simulink model "arq11"  (R2013a)
settings: Solver=ode45  StartTime=0.0  StopTime=Tsim  RelTol=1e-3
values from neighbouring files (symbols this model uses):
  D = 4.1019    [load_variables.m]    (also in matlab.mat; matlab2.mat; matlab_workspace.mat)
  dist = 0    [Ensaios_artigo.m]    (also in load_variables.m = 5; matlab.mat = 5; matlab2.mat = 5; matlab_workspace.mat = 5)
  gain_reduce = 0.9    [Ensaios_artigo.m]
  I = 0.0044    [load_variables.m]    (also in matlab.mat; matlab2.mat; matlab_workspace.mat)
  P = 0.3105    [load_variables.m]    (also in matlab.mat; matlab2.mat; matlab_workspace.mat)
  ref = 10    [Ensaios_artigo.m]    (also in load_variables.m; matlab.mat; matlab2.mat; matlab_workspace.mat)
  Tdist = 0    [Ensaios_artigo.m]    (also in RenameVar.m = Tstep; matlab.mat = 1200; matlab2.mat = 1200; matlab_workspace.mat = 1400)
  Tdistdown = 0    [Ensaios_artigo.m]    (also in RenameVar.m = Tstepdown; matlab.mat = 1800; matlab2.mat = 1800; matlab_workspace.mat = 1800)
  Tref = 700    [Ensaios_artigo.m]    (also in load_variables.m = 800; matlab.mat = 600; matlab2.mat = 600; matlab_workspace.mat)
  Trefdown = Tref*2    (= 1400)    [Ensaios_artigo.m]    (also in load_variables.m = 2420; matlab.mat = 2400; matlab2.mat = 2400; matlab_workspace.mat = 2500)
  Ts = 5    [load_variables.m]    (also in matlab.mat; matlab2.mat; matlab_workspace.mat)
  Tsim = Tref+Trefdown    (= 2100)    [Ensaios_artigo.m]    (also in load_variables.m = 3220; matlab.mat = 800; matlab2.mat = 800; matlab_workspace.mat = 3200)
undefined symbols (not defined in the file): sigma_n, Td
libraries: cstblocks x5, opclib x3, simulink x2, commchan3 x1
settings Model: Creator=didaticontrol  LastModifiedBy=didaticontrol

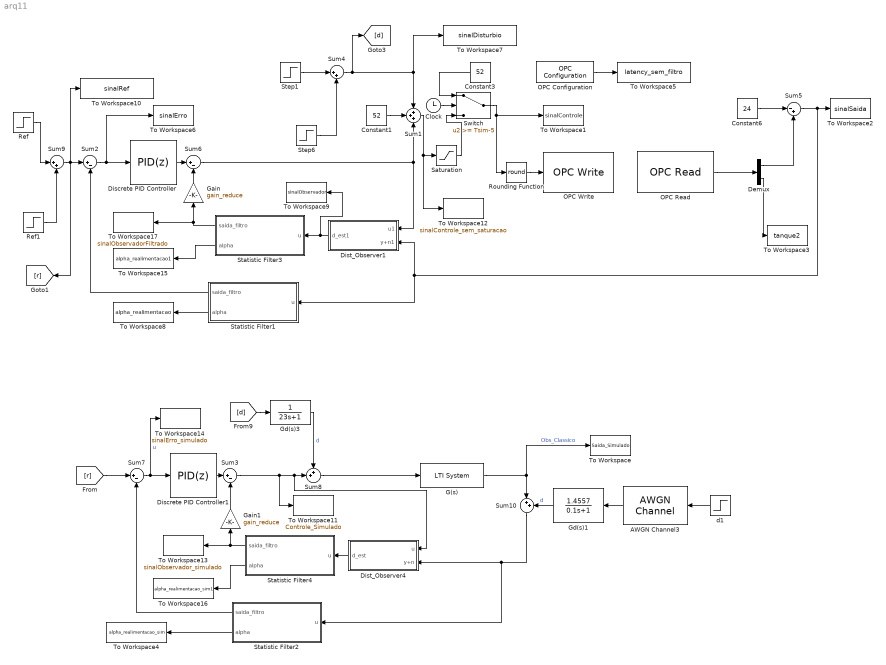
== system arq11 ==
  AWGN Channel3 : commchan3/AWGN Channel  InputProcessing=Columns as channels (frame based)  seed=67  noiseMode=Variance from mask  EbNodB=10  EsNodB=10  SNRdB=10  bitsPerSym=1  Ps=1  Tsym=1  variance=var_ruido
  Clock : Clock
  Constant1 : Constant  Value=52
  Constant3 : Constant  Value=52
  Constant6 : Constant  Value=24
  Demux : Demux  Outputs=2
  Discrete PID Controller : simulink/Continuous/PID Controller  Controller=PID  TimeDomain=Discrete-time  SampleTime=Ts  IntegratorMethod=Forward Euler  FilterMethod=Forward Euler  Form=Parallel  P=P  I=I  D=D  N=0  InitialConditionSource=internal  InitialConditionForIntegrator=0  InitialConditionForFilter=0  ExternalReset=none  LimitOutput=off  UpperSaturationLimit=inf  LowerSaturationLimit=-inf  LinearizeAsGain=off  AntiWindupMode=none  Kb=1  TrackingMode=off  Kt=1  PParamMin=[]  PParamMax=[]  IParamMin=[]  IParamMax=[]  DParamMin=[]  DParamMax=[]  NParamMin=[]  NParamMax=[]  KbParamMin=[]  KbParamMax=[]  KtParamMin=[]  KtParamMax=[]  POutMin=[]  POutMax=[]  IOutMin=[]  IOutMax=[]  DOutMin=[]  DOutMax=[]  NOutMin=[]  NOutMax=[]  KbOutMin=[]  KbOutMax=[]  KtOutMin=[]  KtOutMax=[]  IntegratorOutMin=[]  IntegratorOutMax=[]  FilterOutMin=[]  FilterOutMax=[]  SumOutMin=[]  SumOutMax=[]  SumI1OutMin=[]  SumI1OutMax=[]  SumI2OutMin=[]  SumI2OutMax=[]  SumI3OutMin=[]  SumI3OutMax=[]  SumDOutMin=[]  SumDOutMax=[]  SaturationOutMin=[]  SaturationOutMax=[]  IntegratorContinuousStateAttributes=''  IntegratorStateMustResolveToSignalObject=off  IntegratorRTWStateStorageClass=Auto  FilterContinuousStateAttributes=''  FilterStateMustResolveToSignalObject=off  FilterRTWStateStorageClass=Auto
  Discrete PID Controller1 : simulink/Continuous/PID Controller  Controller=PID  TimeDomain=Discrete-time  SampleTime=Ts  IntegratorMethod=Forward Euler  FilterMethod=Forward Euler  Form=Parallel  P=P  I=I  D=D  N=0  InitialConditionSource=internal  InitialConditionForIntegrator=0  InitialConditionForFilter=0  ExternalReset=none  LimitOutput=off  UpperSaturationLimit=inf  LowerSaturationLimit=-inf  LinearizeAsGain=off  AntiWindupMode=none  Kb=1  TrackingMode=off  Kt=1  PParamMin=[]  PParamMax=[]  IParamMin=[]  IParamMax=[]  DParamMin=[]  DParamMax=[]  NParamMin=[]  NParamMax=[]  KbParamMin=[]  KbParamMax=[]  KtParamMin=[]  KtParamMax=[]  POutMin=[]  POutMax=[]  IOutMin=[]  IOutMax=[]  DOutMin=[]  DOutMax=[]  NOutMin=[]  NOutMax=[]  KbOutMin=[]  KbOutMax=[]  KtOutMin=[]  KtOutMax=[]  IntegratorOutMin=[]  IntegratorOutMax=[]  FilterOutMin=[]  FilterOutMax=[]  SumOutMin=[]  SumOutMax=[]  SumI1OutMin=[]  SumI1OutMax=[]  SumI2OutMin=[]  SumI2OutMax=[]  SumI3OutMin=[]  SumI3OutMax=[]  SumDOutMin=[]  SumDOutMax=[]  SaturationOutMin=[]  SaturationOutMax=[]  IntegratorContinuousStateAttributes=''  IntegratorStateMustResolveToSignalObject=off  IntegratorRTWStateStorageClass=Auto  FilterContinuousStateAttributes=''  FilterStateMustResolveToSignalObject=off  FilterRTWStateStorageClass=Auto
  Dist_Observer1 : Subsystem  mask{Td=Td}
      mask prompts: Td "Filter time cte (Td)"
  Dist_Observer4 : Subsystem  mask{Td=Td}
      mask prompts: Td "Filter time cte (Td)"
  G(s) : cstblocks/LTI System  sys=Gs  IC=[]
  Gain : Gain  Gain=gain_reduce
  Gain1 : Gain  Gain=gain_reduce
  Gd(s)1 : TransferFcn  Numerator=1.4557  Denominator=[0.1 1]
  Gd(s)3 : TransferFcn  Numerator=1  Denominator=[23 1]
  OPC Configuration : opclib/OPC Configuration  opcServers=143.106.123.105/BR.OPC.Server_AR/10  errMissingItems=Error  errReadWrite=Warn  errShutdown=Error  errRTViolation=Warn  rtEnable=on  speedup=1  showLatency=on  beingUsed=on
  OPC Read : opclib/OPC Read  serverHost=143.106.123.105  serverID=BR.OPC.Server_AR  itemIDs=PTQ4_corrigido, PTQ2_corrigido  readMode=Synchronous (cache)  dataType=double  updateRate=5  showQual=off  showTS=off  tsMode=Seconds since start
  OPC Write : opclib/OPC Write  serverHost=143.106.123.105  serverID=BR.OPC.Server_AR  itemIDs=Bomba2  writeMode=Synchronous  updateRate=-1
  Ref : Step  Time=Tref  After=ref  SampleTime=0
  Ref1 : Step  Time=Trefdown  After=-ref  SampleTime=0
  Rounding Function : Rounding  Operator=round
  Saturation : Saturate  UpperLimit=80  LowerLimit=0
  Statistic Filter1 : MATLAB Function  TreatAsAtomicUnit=on  mask{std_dev=sigma_n}
      mask prompts: std_dev "Noise Std Deviation (std_dev)"
  Statistic Filter2 : MATLAB Function  TreatAsAtomicUnit=on  mask{std_dev=sigma_n}
      mask prompts: std_dev "Noise Std Deviation (std_dev)"
  Statistic Filter3 : MATLAB Function  TreatAsAtomicUnit=on  mask{std_dev=2*sigma_n}
      mask prompts: std_dev "Noise Std Deviation (std_dev)"
  Statistic Filter4 : MATLAB Function  TreatAsAtomicUnit=on  mask{std_dev=2*sigma_n}
      mask prompts: std_dev "Noise Std Deviation (std_dev)"
  Step1 : Step  Time=Tdist  After=dist  SampleTime=0
  Step6 : Step  Time=Tdistdown  After=-dist  SampleTime=0
  Sum1 : Sum  Inputs=+++
  Sum10 : Sum  Inputs=|++
  Sum{2..3,6..7} (4 alike) : Sum  Inputs=|+-
  Sum4 : Sum  Inputs=|++
  Sum5 : Sum  Inputs=|-+
  Sum8 : Sum  Inputs=++|
  Sum9 : Sum  Inputs=|++
  Switch : Switch  Threshold=Tsim-5
  To Workspace : ToWorkspace  VariableName=Saida_Simulado  SampleTime=-1  SaveFormat=Timeseries
  To Workspace1 : ToWorkspace  VariableName=sinalControle  SampleTime=Ts  SaveFormat=Timeseries
  To Workspace10 : ToWorkspace  VariableName=sinalRef  SampleTime=Ts  SaveFormat=Timeseries
  To Workspace11 : ToWorkspace  VariableName=Controle_Simulado  SampleTime=-1  SaveFormat=Timeseries
  To Workspace12 : ToWorkspace  VariableName=sinalControle_sem_saturacao  SampleTime=Ts  SaveFormat=Timeseries
  To Workspace13 : ToWorkspace  VariableName=sinalObservador_simulado  SampleTime=Ts  SaveFormat=Timeseries
  To Workspace14 : ToWorkspace  VariableName=sinalErro_simulado  SampleTime=Ts  SaveFormat=Timeseries
  To Workspace15 : ToWorkspace  VariableName=alpha_realimentacao1  SampleTime=-1  SaveFormat=Timeseries
  To Workspace16 : ToWorkspace  VariableName=alpha_realimentacao_sim1  SampleTime=-1  SaveFormat=Timeseries
  To Workspace17 : ToWorkspace  VariableName=sinalObservadorFiltrado  SampleTime=Ts  SaveFormat=Timeseries
  To Workspace2 : ToWorkspace  VariableName=sinalSaida  SampleTime=Ts  SaveFormat=Timeseries
  To Workspace3 : ToWorkspace  VariableName=tanque2  SampleTime=Ts  SaveFormat=Timeseries
  To Workspace4 : ToWorkspace  VariableName=alpha_realimentacao_sim  SampleTime=-1  SaveFormat=Timeseries
  To Workspace5 : ToWorkspace  VariableName=latency_sem_filtro  SampleTime=Ts  SaveFormat=Timeseries
  To Workspace6 : ToWorkspace  VariableName=sinalErro  SampleTime=Ts  SaveFormat=Timeseries
  To Workspace7 : ToWorkspace  VariableName=sinalDisturbio  SampleTime=Ts  SaveFormat=Timeseries
  To Workspace8 : ToWorkspace  VariableName=alpha_realimentacao  SampleTime=-1  SaveFormat=Timeseries
  To Workspace9 : ToWorkspace  VariableName=sinalObservador  SampleTime=Ts  SaveFormat=Timeseries
  d1 : Step  Time=0  After=0  SampleTime=Ts
  wires:
  Sum10/1 -> Dist_Observer4/2(y+n), Statistic Filter2/1(u)
  Sum2/1 -> To Workspace6/1, Discrete PID Controller/1
  Constant6/1 -> Sum5/1
  OPC Read/1 -> Demux/1
  Demux/1 -> Sum5/2
  Demux/2 -> To Workspace3/1
  OPC Configuration/1 -> To Workspace5/1
  Step6/1 -> Sum4/2
  Step1/1 -> Sum4/1
  Constant1/1 -> Sum1/2
  Rounding Function/1 -> OPC Write/1
  Sum5/1 -> Statistic Filter1/1(u), Dist_Observer1/2(y+n1), To Workspace2/1
  Discrete PID Controller/1 -> Sum6/1
  Sum6/1 -> Dist_Observer1/1(u1), Sum1/3
  Ref/1 -> Sum9/1
  Ref1/1 -> Sum9/2
  Clock/1 -> Switch/2
  Constant3/1 -> Switch/1
  Switch/1 -> Rounding Function/1, To Workspace1/1
  Saturation/1 -> Switch/3
  [r] -> Sum7/1
  Sum8/1 -> G(s)/1
  G(s)/1 -> To Workspace/1, Sum10/1  "Obs_Classico"
  [d] -> Gd(s)3/1
  Gd(s)3/1 -> Sum8/1  "d"
  Sum7/1 -> To Workspace14/1, Discrete PID Controller1/1  "u"
  d1/1 -> AWGN Channel3/1
  AWGN Channel3/1 -> Gd(s)1/1
  Gd(s)1/1 -> Sum10/2  "d"
  Discrete PID Controller1/1 -> Sum3/1
  Sum3/1 -> To Workspace11/1, Dist_Observer4/1(u), Sum8/2
  Sum4/1 -> To Workspace7/1, Sum1/1, [d]
  Sum9/1 -> [r], Sum2/1, To Workspace10/1
  Sum1/1 -> To Workspace12/1, Saturation/1
  Statistic Filter1/2(alpha) -> To Workspace8/1
  Statistic Filter1/1(saida_filtro) -> Sum2/2
  Dist_Observer1/1(d_est1) -> To Workspace9/1, Statistic Filter3/1(u)
  Statistic Filter3/1(saida_filtro) -> To Workspace17/1, Gain/1
  Statistic Filter3/2(alpha) -> To Workspace15/1
  Statistic Filter2/2(alpha) -> To Workspace4/1
  Statistic Filter2/1(saida_filtro) -> Sum7/2
  Statistic Filter4/2(alpha) -> To Workspace16/1
  Dist_Observer4/1(d_est) -> Statistic Filter4/1(u)
  Statistic Filter4/1(saida_filtro) -> To Workspace13/1, Gain1/1
  Gain/1 -> Sum6/2
  Gain1/1 -> Sum3/2

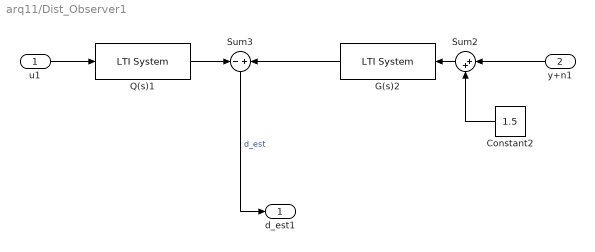
== system arq11/Dist_Observer1 ==
  u1 : Inport
  y+n1 : Inport  Port=2
  Constant2 : Constant  Value=1.5
  G(s)2 : cstblocks/LTI System  sys=G_inv_Q  IC=[]
  Q(s)1 : cstblocks/LTI System  sys=Qs  IC=[]
  Sum2 : Sum  Inputs=|++
  Sum3 : Sum  Inputs=-|+
  d_est1 : Outport
  wires:
  Q(s)1/1 -> Sum3/1
  Sum3/1 -> d_est1/1  "d_est"
  Sum2/1 -> G(s)2/1
  u1/1 -> Q(s)1/1
  Constant2/1 -> Sum2/2
  y+n1/1 -> Sum2/1
  G(s)2/1 -> Sum3/2

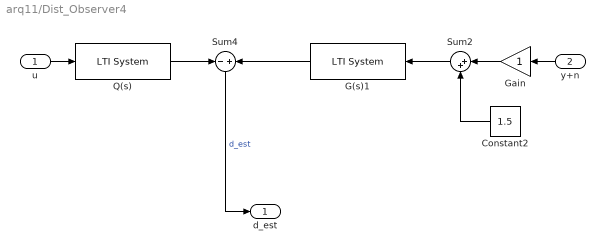
== system arq11/Dist_Observer4 ==
  u : Inport
  y+n : Inport  Port=2
  Constant2 : Constant  Value=1.5
  G(s)1 : cstblocks/LTI System  sys=G_inv_Q  IC=[]
  Gain : Gain
  Q(s) : cstblocks/LTI System  sys=Qs  IC=[]
  Sum2 : Sum  Inputs=|++
  Sum4 : Sum  Inputs=-|+
  d_est : Outport
  wires:
  Q(s)/1 -> Sum4/1
  Sum4/1 -> d_est/1  "d_est"
  u/1 -> Q(s)/1
  G(s)1/1 -> Sum4/2
  Constant2/1 -> Sum2/2
  Gain/1 -> Sum2/1
  Sum2/1 -> G(s)1/1
  y+n/1 -> Gain/1

== matlab function arq11/Statistic Filter2 ==
  settings: updateMethod=DISCRETE
  data: u input; saida_filtro output; std_dev parameter; alpha output
%Autor: Lucas Moura Gomes
%Filtro estatístico.

function [saida_filtro, alpha]  = filtroPID( u, std_dev)
    persistent x_ant;
    persistent alpha_orig;
    
    if isempty(x_ant)
        x_ant = 0;
        Ts = 0.01; %sampling time
        tf = 2; %continuous time cte.
        alpha_orig = 1 - exp(-1/tf * Ts); %c2d filter
    end
    
    alpha = erf(abs(x_ant - u)/(sqrt(2)*2*std_dev));
    
    if alpha > 1
        alpha = 1;
    end
    
    %up = 1.1; %upper bound 10%
    %alpha = alpha * alpha_orig * up;
    
    saida_filtro = (1-alpha)*x_ant + alpha*u;
    
    x_ant = saida_filtro;
end

%Autor: Lucas Moura Gomes
%Filtro estatístico.
% 
% function [saida_filtro, alpha] = filtroPID( u, erro_tipico_medicao, Tf  )
% 	
%     persistent x_ant;
%     
%     if isempty(x_ant)
%         x_ant = 0;
%     end
%     
%     Tf = Tf/1.5;
%     a_Tf = 1 - exp(-1/Tf * 5);
%     
%     alpha = erf(abs(x_ant - u)/(sqrt(2)*2*erro_tipico_medicao));
%     
%     if alpha > 1 
%         alpha = 1;
%     end;
%     
%     saida_filtro = (1-alpha)*x_ant + alpha*u;
% 
%     x_ant = saida_filtro;
%         
% 
%     saida_filtro = x_ant;
% 
%     
% end

== matlab function arq11/Statistic Filter1 ==
  settings: updateMethod=DISCRETE
  data: u input; saida_filtro output; std_dev parameter; alpha output
%Autor: Lucas Moura Gomes
%Filtro estatístico.

function [saida_filtro, alpha]  = filtroPID( u, std_dev)
    persistent x_ant;
    persistent alpha_orig;
    
    if isempty(x_ant)
        x_ant = 0;
        Ts = 0.01; %sampling time
        tf = 2; %continuous time cte.
        alpha_orig = 1 - exp(-1/tf * Ts); %c2d filter
    end
    
    alpha = erf(abs(x_ant - u)/(sqrt(2)*2*std_dev));
    
    if alpha > 1
        alpha = 1;
    end
    
    %up = 1.1; %upper bound 10%
    %alpha = alpha * alpha_orig * up;
    
    saida_filtro = (1-alpha)*x_ant + alpha*u;
    
    x_ant = saida_filtro;
end

%Autor: Lucas Moura Gomes
%Filtro estatístico.
% 
% function [saida_filtro, alpha] = filtroPID( u, erro_tipico_medicao, Tf  )
% 	
%     persistent x_ant;
%     
%     if isempty(x_ant)
%         x_ant = 0;
%     end
%     
%     Tf = Tf/1.5;
%     a_Tf = 1 - exp(-1/Tf * 5);
%     
%     alpha = erf(abs(x_ant - u)/(sqrt(2)*2*erro_tipico_medicao));
%     
%     if alpha > 1 
%         alpha = 1;
%     end;
%     
%     saida_filtro = (1-alpha)*x_ant + alpha*u;
% 
%     x_ant = saida_filtro;
%         
% 
%     saida_filtro = x_ant;
% 
%     
% end

== matlab function arq11/Statistic Filter3 ==
  settings: updateMethod=DISCRETE
  data: u input; saida_filtro output; std_dev parameter; alpha output
%Autor: Lucas Moura Gomes
%Filtro estatístico.

function [saida_filtro, alpha]  = filtroPID( u, std_dev)
    persistent x_ant;
    persistent alpha_orig;
    
    if isempty(x_ant)
        x_ant = 0;
        Ts = 0.01; %sampling time
        tf = 2; %continuous time cte.
        alpha_orig = 1 - exp(-1/tf * Ts); %c2d filter
    end
    
    alpha = erf(abs(x_ant - u)/(sqrt(2)*2*std_dev));
    
    if alpha > 1
        alpha = 1;
    end
    
    %up = 1.1; %upper bound 10%
    %alpha = alpha * alpha_orig * up;
    
    saida_filtro = (1-alpha)*x_ant + alpha*u;
    
    x_ant = saida_filtro;
end

%Autor: Lucas Moura Gomes
%Filtro estatístico.
% 
% function [saida_filtro, alpha] = filtroPID( u, erro_tipico_medicao, Tf  )
% 	
%     persistent x_ant;
%     
%     if isempty(x_ant)
%         x_ant = 0;
%     end
%     
%     Tf = Tf/1.5;
%     a_Tf = 1 - exp(-1/Tf * 5);
%     
%     alpha = erf(abs(x_ant - u)/(sqrt(2)*2*erro_tipico_medicao));
%     
%     if alpha > 1 
%         alpha = 1;
%     end;
%     
%     saida_filtro = (1-alpha)*x_ant + alpha*u;
% 
%     x_ant = saida_filtro;
%         
% 
%     saida_filtro = x_ant;
% 
%     
% end

== matlab function arq11/Statistic Filter4 ==
  settings: updateMethod=DISCRETE
  data: u input; saida_filtro output; std_dev parameter; alpha output
%Autor: Lucas Moura Gomes
%Filtro estatístico.

function [saida_filtro, alpha]  = filtroPID( u, std_dev)
    persistent x_ant;
    persistent alpha_orig;
    
    if isempty(x_ant)
        x_ant = 0;
        Ts = 0.01; %sampling time
        tf = 2; %continuous time cte.
        alpha_orig = 1 - exp(-1/tf * Ts); %c2d filter
    end
    
    alpha = erf(abs(x_ant - u)/(sqrt(2)*2*std_dev));
    
    if alpha > 1
        alpha = 1;
    end
    
    %up = 1.1; %upper bound 10%
    %alpha = alpha * alpha_orig * up;
    
    saida_filtro = (1-alpha)*x_ant + alpha*u;
    
    x_ant = saida_filtro;
end

%Autor: Lucas Moura Gomes
%Filtro estatístico.
% 
% function [saida_filtro, alpha] = filtroPID( u, erro_tipico_medicao, Tf  )
% 	
%     persistent x_ant;
%     
%     if isempty(x_ant)
%         x_ant = 0;
%     end
%     
%     Tf = Tf/1.5;
%     a_Tf = 1 - exp(-1/Tf * 5);
%     
%     alpha = erf(abs(x_ant - u)/(sqrt(2)*2*erro_tipico_medicao));
%     
%     if alpha > 1 
%         alpha = 1;
%     end;
%     
%     saida_filtro = (1-alpha)*x_ant + alpha*u;
% 
%     x_ant = saida_filtro;
%         
% 
%     saida_filtro = x_ant;
% 
%     
% end
